simulink model "keyboardTask"  (R2012b)
settings: Solver=FixedStepDiscrete  StartTime=0.0  StopTime=10.0  FixedStep=0.001  RelTol=1e-3
undefined symbols (not defined in the file or in its folder): acquireMethods, autoplayMovementDuration, autoplayReactionTime, autoplayRotationDuration, autoplayRotationStart, centerOffset, clickPercentage, clickRefractoryPeriod, clickTargetColor, clickTargetHoverColor, cuedText, cuedTextLength, cumulativeDwell, cursorColorClick, cursorColorClosed, cursorColorOpen, cursorDiameter, cursorNeuralColor, cursorNonneuralColor, delayOrder, displayObject, displayShape, displayShape_1, displayShape_10, displayShape_11, displayShape_12, displayShape_13, displayShape_14, displayShape_15, displayShape_16, displayShape_17, displayShape_18, displayShape_19, displayShape_2, displayShape_3, displayShape_4, displayShape_5, displayShape_6, displayShape_7, displayShape_8, displayShape_9, dwellRefractoryPeriod, errorAssistAxis, errorAssistR, errorAssistTheta, expRandBinSize, expRandMax, expRandMin, expRandMu, failOnLiftoff, failurePenalty, falseClickFails, fingerPositionTolerance, fixedSeqMode, gain, gloveBias, gloveLPDenominator, gloveLPNumerator, gloveNonlinearCorrection, gloveXCorrection ... (+327)
(part 1 of 2)
settings Model: Creator=gilja  LastModifiedBy=NPTL
settings SolverCC: EnableConcurrentExecution=on  ConcurrentTasks=on
settings DataIOCC: SaveOutput=off  SignalLogging=off  SaveTime=off
settings OptimizationCC: InlineParams=on  InlineInvariantSignals=on  EnhancedBackFolding=on  EfficientFloat2IntCast=on  SimCompilerOptimization=On
settings DebuggingCC: UnderspecifiedInitializationDetection=Simplified
settings HardwareCC: ProdIntDivRoundTo=Zero  ProdEndianess=LittleEndian  ProdHWDeviceType=Generic->32-bit x86 compatible
settings RTWCC: SystemTargetFile=xpctarget.tlc  TemplateMakefile=xpc_default_tmf  Description=xPC Target  ProcessScript=xpctarget_make_rtw_hook  RTWCompilerOptimization=On
settings CodeAppCC: MaxIdLength=62
settings xpcTargetCC: TargetFcnLib=ansi_tfl_table_tmw.mat  CodeReplacementLibrary=XPC_BLAS  ParMdlRefBuildCompliant=on  ConcurrentExecutionCompliant=on  CombineSignalStateStructs=off  GRTInterface=on  xPCTaskExecutionProfile=on  xPCRL32EventNumber=5000  xPCisDownloadable=off  xPCLoadParamSetFile=off  xPCConcurrentTasks=off  xPCEnableSFAnimation=off

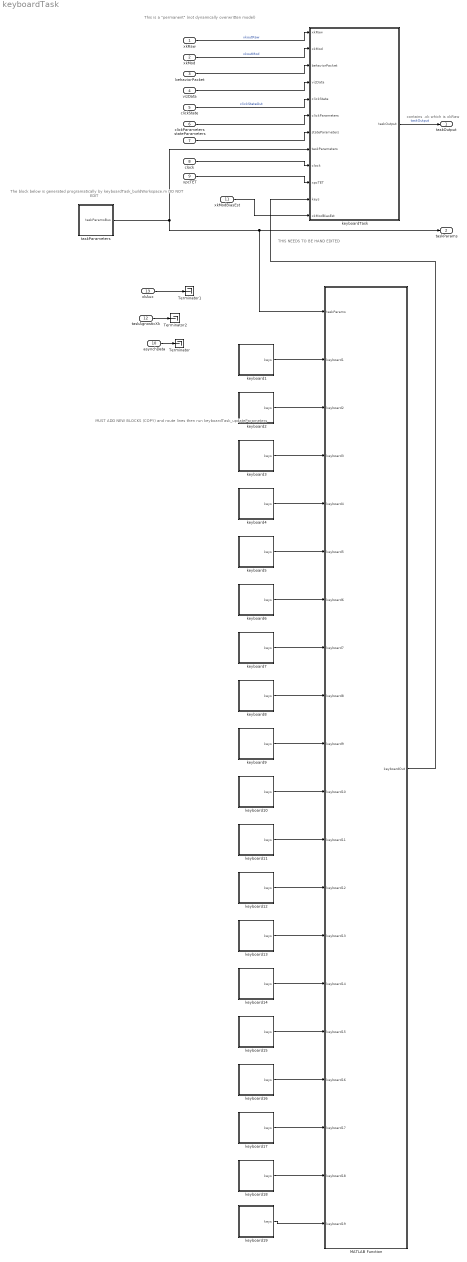
== system keyboardTask ==
  note: MUST ADD NEW BLOCKS (COPY)
      | and route lines
      | then run keyboardTask_updateParameters
  note: THIS NEEDS TO BE HAND EDITED
  note: contains .xk which is xkRaw
  note: The block below is generated programatically
      | by keyboardTask_buildWorkspace.m
      | DO NOT EDIT
  note: This is a "permanent" (not dynamically overwritten model)
  xkRaw : Inport  OutDataTypeStr=double  PortDimensions=[double(xkConstants.NUM_STATE_DIMENSIONS),1]  SampleTime=[0.001,0]
  xkMod : Inport  Port=2  OutDataTypeStr=double  PortDimensions=[double(xkConstants.NUM_STATE_DIMENSIONS),1]  SampleTime=[0.001,0]
  behaviorPacket : Inport  Port=3  OutDataTypeStr=Bus: behaviorPacketBus  SampleTime=[0.001,0]
  vizData : Inport  Port=4  OutDataTypeStr=Bus: peripheralData  SampleTime=[0.001,0]
  clickState : Inport  Port=5  OutDataTypeStr=uint16  PortDimensions=1  SampleTime=[0.001,0]
  clickParameters : Inport  Port=6  OutDataTypeStr=Bus: clickParametersBus  SampleTime=[0.001,0]
  stateParameters : Inport  Port=7  OutDataTypeStr=Bus: stateParams  SampleTime=[0.001,0]
  clock : Inport  Port=8  OutDataTypeStr=uint32  PortDimensions=1  SampleTime=[0.001,0]
  xpcTET : Inport  Port=9  OutDataTypeStr=double  PortDimensions=1  SampleTime=[0.001,0]
  asynchData : Inport  Port=10  OutDataTypeStr=Bus: peripheralData  SampleTime=[0.001,0]
  xkModBiasEst : Inport  Port=11  OutDataTypeStr=double  PortDimensions=[double(xkConstants.NUM_STATE_DIMENSIONS),1]  SampleTime=[0.001,0]
  taskAgnosticXk : Inport  Port=12  OutDataTypeStr=double  PortDimensions=[double(xkConstants.NUM_STATE_DIMENSIONS),1]  SampleTime=[0.001,0]
  xkAux : Inport  Port=13  OutDataTypeStr=double  PortDimensions=[double(xkConstants.NUM_STATE_DIMENSIONS),1]  SampleTime=[0.001,0]
  MATLAB Function : MATLAB Function  TreatAsAtomicUnit=on
  Terminator : Terminator
  Terminator1 : Terminator
  Terminator2 : Terminator
  keyboard1 : Subsystem
  keyboard10 : Subsystem
  keyboard11 : Subsystem
  keyboard12 : Subsystem
  keyboard13 : Subsystem
  keyboard14 : Subsystem
  keyboard15 : Subsystem
  keyboard16 : Subsystem
  keyboard17 : Subsystem
  keyboard18 : Subsystem
  keyboard19 : Subsystem
  keyboard2 : Subsystem
  keyboard3 : Subsystem
  keyboard4 : Subsystem
  keyboard5 : Subsystem
  keyboard6 : Subsystem
  keyboard7 : Subsystem
  keyboard8 : Subsystem
  keyboard9 : Subsystem
  keyboardTask : MATLAB Function  TreatAsAtomicUnit=on
  taskParameters : Subsystem
  taskOutput : Outport  OutDataTypeStr=Bus: taskOutput  PortDimensions=1  SampleTime=[0.001,0]  BusOutputAsStruct=on
  taskParams : Outport  Port=2  OutDataTypeStr=Bus: taskParamsBus  SampleTime=[0.001,0]
  wires:
  behaviorPacket/1 -> keyboardTask/3(behaviorPacket)
  vizData/1 -> keyboardTask/4(vizData)
  clickState/1 -> keyboardTask/5(clickState)  "clickStateOut"
  clickParameters/1 -> keyboardTask/6(clickParameters)
  clock/1 -> keyboardTask/9(clock)
  xpcTET/1 -> keyboardTask/10(xpcTET)
  keyboardTask/1(taskOutput) -> taskOutput/1  "taskOutput"
  stateParameters/1 -> keyboardTask/7(stateParameters)
  taskParameters/1(taskParamsBus) -> MATLAB Function/1(taskParams), taskParams/1, keyboardTask/8(taskParameters)
  MATLAB Function/1(keyboardOut) -> keyboardTask/11(keys)
  asynchData/1 -> Terminator/1
  xkRaw/1 -> keyboardTask/1(xkRaw)  "xkoutRaw"
  xkMod/1 -> keyboardTask/2(xkMod)  "xkoutMod"
  keyboard4/1(keys) -> MATLAB Function/5(keyboard4)
  keyboard3/1(keys) -> MATLAB Function/4(keyboard3)
  keyboard5/1(keys) -> MATLAB Function/6(keyboard5)
  keyboard2/1(keys) -> MATLAB Function/3(keyboard2)
  keyboard6/1(keys) -> MATLAB Function/7(keyboard6)
  keyboard7/1(keys) -> MATLAB Function/8(keyboard7)
  keyboard1/1(keys) -> MATLAB Function/2(keyboard1)
  keyboard8/1(keys) -> MATLAB Function/9(keyboard8)
  keyboard9/1(keys) -> MATLAB Function/10(keyboard9)
  keyboard10/1(keys) -> MATLAB Function/11(keyboard10)
  keyboard11/1(keys) -> MATLAB Function/12(keyboard11)
  keyboard12/1(keys) -> MATLAB Function/13(keyboard12)
  keyboard13/1(keys) -> MATLAB Function/14(keyboard13)
  keyboard14/1(keys) -> MATLAB Function/15(keyboard14)
  keyboard15/1(keys) -> MATLAB Function/16(keyboard15)
  keyboard16/1(keys) -> MATLAB Function/17(keyboard16)
  keyboard17/1(keys) -> MATLAB Function/18(keyboard17)
  keyboard18/1(keys) -> MATLAB Function/19(keyboard18)
  keyboard19/1(keys) -> MATLAB Function/20(keyboard19)
  xkAux/1 -> Terminator1/1
  taskAgnosticXk/1 -> Terminator2/1
  xkModBiasEst/1 -> keyboardTask/12(xkModBiasEst)

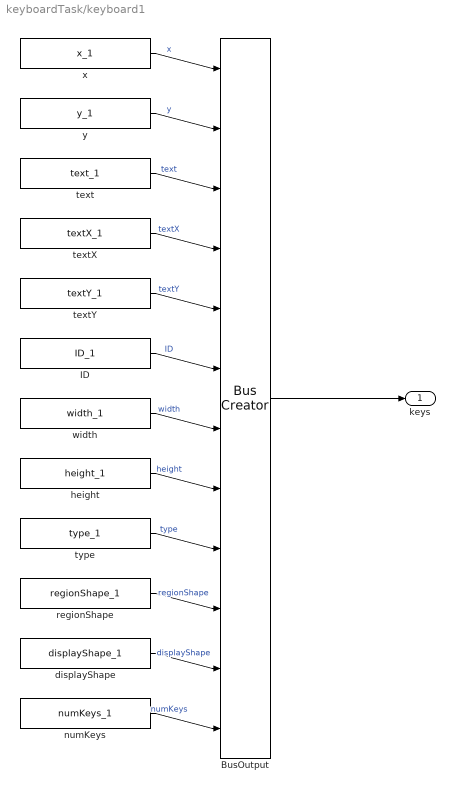
== system keyboardTask/keyboard1 ==
  BusOutput : BusCreator  Inputs=x,y,text,textX,textY,ID,width,height,type,regionShape,displayShape,numKeys  OutDataTypeStr=Bus: keysParamsBus
  ID : Constant  Value=ID_1
  displayShape : Constant  Value=displayShape_1
  height : Constant  Value=height_1
  numKeys : Constant  Value=numKeys_1
  regionShape : Constant  Value=regionShape_1
  text : Constant  Value=text_1
  textX : Constant  Value=textX_1
  textY : Constant  Value=textY_1
  type : Constant  Value=type_1
  width : Constant  Value=width_1
  x : Constant  Value=x_1
  y : Constant  Value=y_1
  keys : Outport
  wires:
  x/1 -> BusOutput/1  "x"
  y/1 -> BusOutput/2  "y"
  text/1 -> BusOutput/3  "text"
  textX/1 -> BusOutput/4  "textX"
  textY/1 -> BusOutput/5  "textY"
  ID/1 -> BusOutput/6  "ID"
  width/1 -> BusOutput/7  "width"
  height/1 -> BusOutput/8  "height"
  type/1 -> BusOutput/9  "type"
  regionShape/1 -> BusOutput/10  "regionShape"
  displayShape/1 -> BusOutput/11  "displayShape"
  numKeys/1 -> BusOutput/12  "numKeys"
  BusOutput/1 -> keys/1

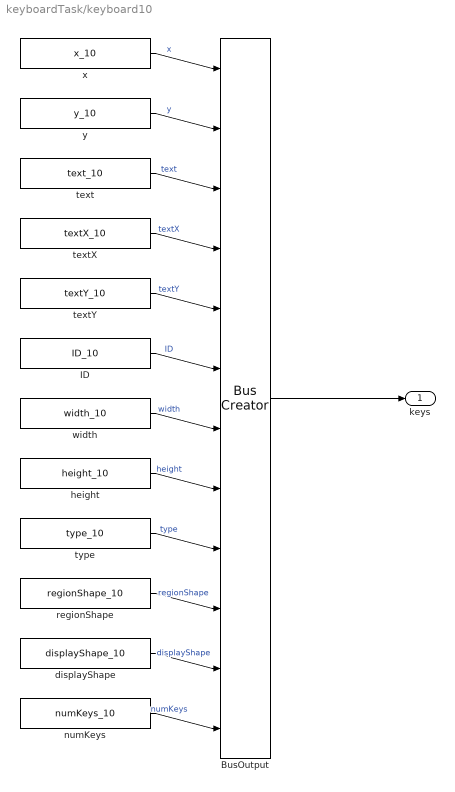
== system keyboardTask/keyboard10 ==
  BusOutput : BusCreator  Inputs=x,y,text,textX,textY,ID,width,height,type,regionShape,displayShape,numKeys  OutDataTypeStr=Bus: keysParamsBus
  ID : Constant  Value=ID_10
  displayShape : Constant  Value=displayShape_10
  height : Constant  Value=height_10
  numKeys : Constant  Value=numKeys_10
  regionShape : Constant  Value=regionShape_10
  text : Constant  Value=text_10
  textX : Constant  Value=textX_10
  textY : Constant  Value=textY_10
  type : Constant  Value=type_10
  width : Constant  Value=width_10
  x : Constant  Value=x_10
  y : Constant  Value=y_10
  keys : Outport  OutDataTypeStr=Bus: keysParamsBus
  wires:
  x/1 -> BusOutput/1  "x"
  y/1 -> BusOutput/2  "y"
  text/1 -> BusOutput/3  "text"
  textX/1 -> BusOutput/4  "textX"
  textY/1 -> BusOutput/5  "textY"
  ID/1 -> BusOutput/6  "ID"
  width/1 -> BusOutput/7  "width"
  height/1 -> BusOutput/8  "height"
  type/1 -> BusOutput/9  "type"
  regionShape/1 -> BusOutput/10  "regionShape"
  displayShape/1 -> BusOutput/11  "displayShape"
  numKeys/1 -> BusOutput/12  "numKeys"
  BusOutput/1 -> keys/1

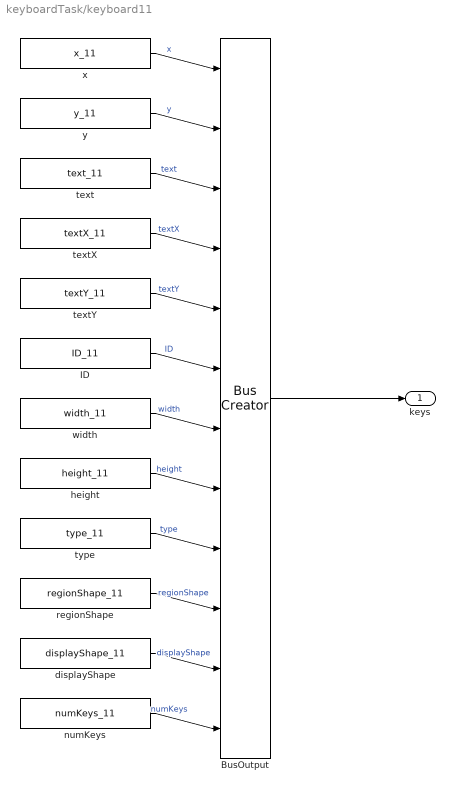
== system keyboardTask/keyboard11 ==
  BusOutput : BusCreator  Inputs=x,y,text,textX,textY,ID,width,height,type,regionShape,displayShape,numKeys  OutDataTypeStr=Bus: keysParamsBus
  ID : Constant  Value=ID_11
  displayShape : Constant  Value=displayShape_11
  height : Constant  Value=height_11
  numKeys : Constant  Value=numKeys_11
  regionShape : Constant  Value=regionShape_11
  text : Constant  Value=text_11
  textX : Constant  Value=textX_11
  textY : Constant  Value=textY_11
  type : Constant  Value=type_11
  width : Constant  Value=width_11
  x : Constant  Value=x_11
  y : Constant  Value=y_11
  keys : Outport  OutDataTypeStr=Bus: keysParamsBus
  wires:
  x/1 -> BusOutput/1  "x"
  y/1 -> BusOutput/2  "y"
  text/1 -> BusOutput/3  "text"
  textX/1 -> BusOutput/4  "textX"
  textY/1 -> BusOutput/5  "textY"
  ID/1 -> BusOutput/6  "ID"
  width/1 -> BusOutput/7  "width"
  height/1 -> BusOutput/8  "height"
  type/1 -> BusOutput/9  "type"
  regionShape/1 -> BusOutput/10  "regionShape"
  displayShape/1 -> BusOutput/11  "displayShape"
  numKeys/1 -> BusOutput/12  "numKeys"
  BusOutput/1 -> keys/1

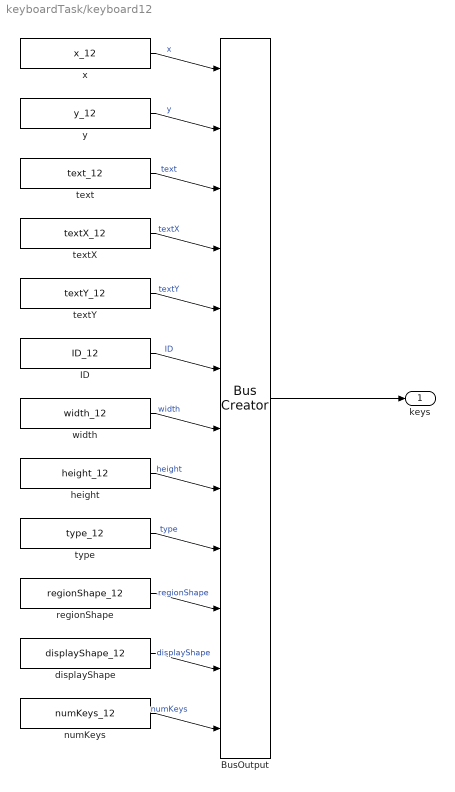
== system keyboardTask/keyboard12 ==
  BusOutput : BusCreator  Inputs=x,y,text,textX,textY,ID,width,height,type,regionShape,displayShape,numKeys  OutDataTypeStr=Bus: keysParamsBus
  ID : Constant  Value=ID_12
  displayShape : Constant  Value=displayShape_12
  height : Constant  Value=height_12
  numKeys : Constant  Value=numKeys_12
  regionShape : Constant  Value=regionShape_12
  text : Constant  Value=text_12
  textX : Constant  Value=textX_12
  textY : Constant  Value=textY_12
  type : Constant  Value=type_12
  width : Constant  Value=width_12
  x : Constant  Value=x_12
  y : Constant  Value=y_12
  keys : Outport  OutDataTypeStr=Bus: keysParamsBus
  wires:
  x/1 -> BusOutput/1  "x"
  y/1 -> BusOutput/2  "y"
  text/1 -> BusOutput/3  "text"
  textX/1 -> BusOutput/4  "textX"
  textY/1 -> BusOutput/5  "textY"
  ID/1 -> BusOutput/6  "ID"
  width/1 -> BusOutput/7  "width"
  height/1 -> BusOutput/8  "height"
  type/1 -> BusOutput/9  "type"
  regionShape/1 -> BusOutput/10  "regionShape"
  displayShape/1 -> BusOutput/11  "displayShape"
  numKeys/1 -> BusOutput/12  "numKeys"
  BusOutput/1 -> keys/1

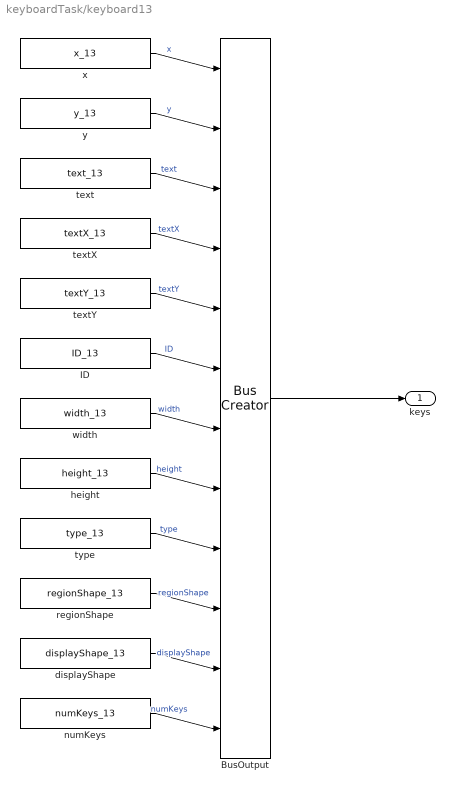
== system keyboardTask/keyboard13 ==
  BusOutput : BusCreator  Inputs=x,y,text,textX,textY,ID,width,height,type,regionShape,displayShape,numKeys  OutDataTypeStr=Bus: keysParamsBus
  ID : Constant  Value=ID_13
  displayShape : Constant  Value=displayShape_13
  height : Constant  Value=height_13
  numKeys : Constant  Value=numKeys_13
  regionShape : Constant  Value=regionShape_13
  text : Constant  Value=text_13
  textX : Constant  Value=textX_13
  textY : Constant  Value=textY_13
  type : Constant  Value=type_13
  width : Constant  Value=width_13
  x : Constant  Value=x_13
  y : Constant  Value=y_13
  keys : Outport  OutDataTypeStr=Bus: keysParamsBus
  wires:
  x/1 -> BusOutput/1  "x"
  y/1 -> BusOutput/2  "y"
  text/1 -> BusOutput/3  "text"
  textX/1 -> BusOutput/4  "textX"
  textY/1 -> BusOutput/5  "textY"
  ID/1 -> BusOutput/6  "ID"
  width/1 -> BusOutput/7  "width"
  height/1 -> BusOutput/8  "height"
  type/1 -> BusOutput/9  "type"
  regionShape/1 -> BusOutput/10  "regionShape"
  displayShape/1 -> BusOutput/11  "displayShape"
  numKeys/1 -> BusOutput/12  "numKeys"
  BusOutput/1 -> keys/1

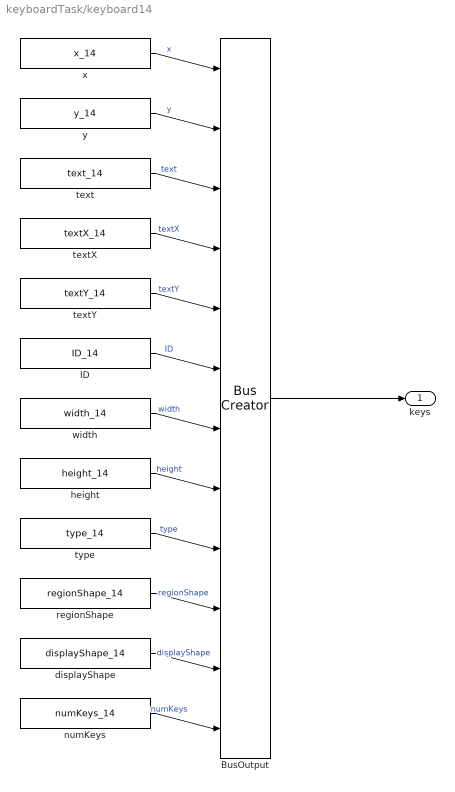
== system keyboardTask/keyboard14 ==
  BusOutput : BusCreator  Inputs=x,y,text,textX,textY,ID,width,height,type,regionShape,displayShape,numKeys  OutDataTypeStr=Bus: keysParamsBus
  ID : Constant  Value=ID_14
  displayShape : Constant  Value=displayShape_14
  height : Constant  Value=height_14
  numKeys : Constant  Value=numKeys_14
  regionShape : Constant  Value=regionShape_14
  text : Constant  Value=text_14
  textX : Constant  Value=textX_14
  textY : Constant  Value=textY_14
  type : Constant  Value=type_14
  width : Constant  Value=width_14
  x : Constant  Value=x_14
  y : Constant  Value=y_14
  keys : Outport  OutDataTypeStr=Bus: keysParamsBus
  wires:
  x/1 -> BusOutput/1  "x"
  y/1 -> BusOutput/2  "y"
  text/1 -> BusOutput/3  "text"
  textX/1 -> BusOutput/4  "textX"
  textY/1 -> BusOutput/5  "textY"
  ID/1 -> BusOutput/6  "ID"
  width/1 -> BusOutput/7  "width"
  height/1 -> BusOutput/8  "height"
  type/1 -> BusOutput/9  "type"
  regionShape/1 -> BusOutput/10  "regionShape"
  displayShape/1 -> BusOutput/11  "displayShape"
  numKeys/1 -> BusOutput/12  "numKeys"
  BusOutput/1 -> keys/1

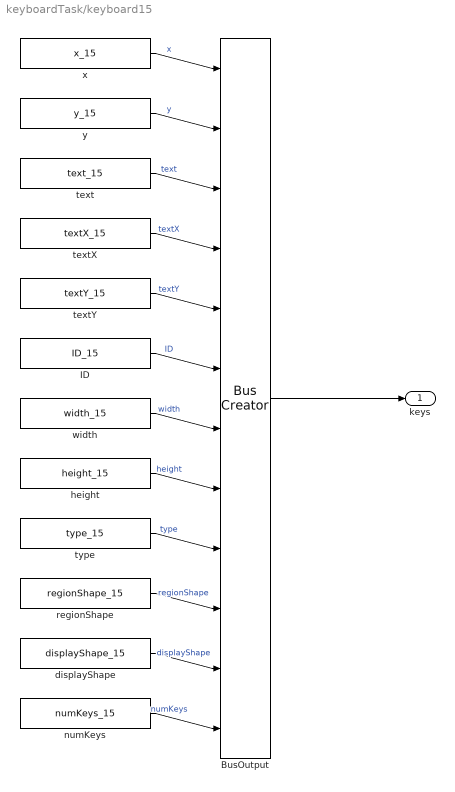
== system keyboardTask/keyboard15 ==
  BusOutput : BusCreator  Inputs=x,y,text,textX,textY,ID,width,height,type,regionShape,displayShape,numKeys  OutDataTypeStr=Bus: keysParamsBus
  ID : Constant  Value=ID_15
  displayShape : Constant  Value=displayShape_15
  height : Constant  Value=height_15
  numKeys : Constant  Value=numKeys_15
  regionShape : Constant  Value=regionShape_15
  text : Constant  Value=text_15
  textX : Constant  Value=textX_15
  textY : Constant  Value=textY_15
  type : Constant  Value=type_15
  width : Constant  Value=width_15
  x : Constant  Value=x_15
  y : Constant  Value=y_15
  keys : Outport  OutDataTypeStr=Bus: keysParamsBus
  wires:
  x/1 -> BusOutput/1  "x"
  y/1 -> BusOutput/2  "y"
  text/1 -> BusOutput/3  "text"
  textX/1 -> BusOutput/4  "textX"
  textY/1 -> BusOutput/5  "textY"
  ID/1 -> BusOutput/6  "ID"
  width/1 -> BusOutput/7  "width"
  height/1 -> BusOutput/8  "height"
  type/1 -> BusOutput/9  "type"
  regionShape/1 -> BusOutput/10  "regionShape"
  displayShape/1 -> BusOutput/11  "displayShape"
  numKeys/1 -> BusOutput/12  "numKeys"
  BusOutput/1 -> keys/1

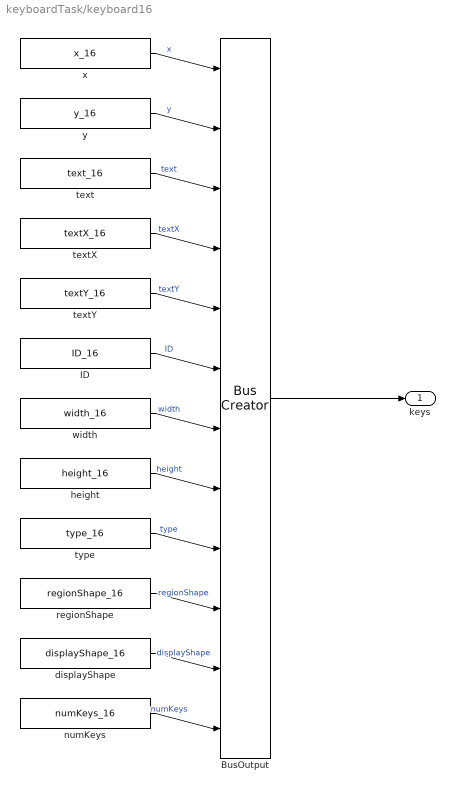
== system keyboardTask/keyboard16 ==
  BusOutput : BusCreator  Inputs=x,y,text,textX,textY,ID,width,height,type,regionShape,displayShape,numKeys  OutDataTypeStr=Bus: keysParamsBus
  ID : Constant  Value=ID_16
  displayShape : Constant  Value=displayShape_16
  height : Constant  Value=height_16
  numKeys : Constant  Value=numKeys_16
  regionShape : Constant  Value=regionShape_16
  text : Constant  Value=text_16
  textX : Constant  Value=textX_16
  textY : Constant  Value=textY_16
  type : Constant  Value=type_16
  width : Constant  Value=width_16
  x : Constant  Value=x_16
  y : Constant  Value=y_16
  keys : Outport  OutDataTypeStr=Bus: keysParamsBus
  wires:
  x/1 -> BusOutput/1  "x"
  y/1 -> BusOutput/2  "y"
  text/1 -> BusOutput/3  "text"
  textX/1 -> BusOutput/4  "textX"
  textY/1 -> BusOutput/5  "textY"
  ID/1 -> BusOutput/6  "ID"
  width/1 -> BusOutput/7  "width"
  height/1 -> BusOutput/8  "height"
  type/1 -> BusOutput/9  "type"
  regionShape/1 -> BusOutput/10  "regionShape"
  displayShape/1 -> BusOutput/11  "displayShape"
  numKeys/1 -> BusOutput/12  "numKeys"
  BusOutput/1 -> keys/1

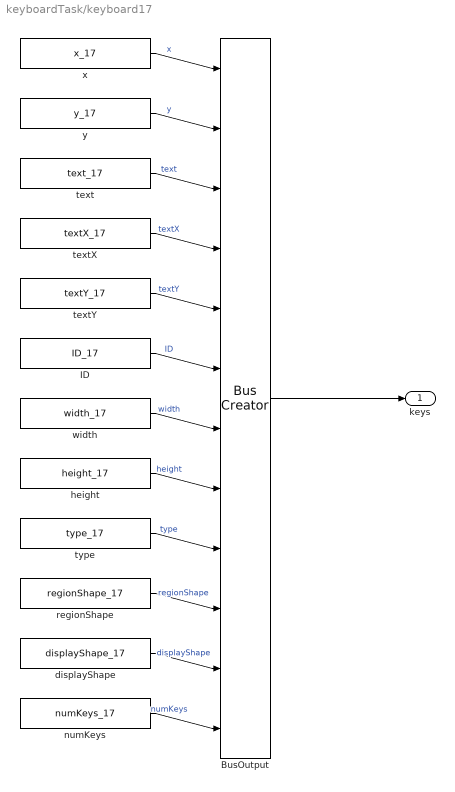
== system keyboardTask/keyboard17 ==
  BusOutput : BusCreator  Inputs=x,y,text,textX,textY,ID,width,height,type,regionShape,displayShape,numKeys  OutDataTypeStr=Bus: keysParamsBus
  ID : Constant  Value=ID_17
  displayShape : Constant  Value=displayShape_17
  height : Constant  Value=height_17
  numKeys : Constant  Value=numKeys_17
  regionShape : Constant  Value=regionShape_17
  text : Constant  Value=text_17
  textX : Constant  Value=textX_17
  textY : Constant  Value=textY_17
  type : Constant  Value=type_17
  width : Constant  Value=width_17
  x : Constant  Value=x_17
  y : Constant  Value=y_17
  keys : Outport  OutDataTypeStr=Bus: keysParamsBus
  wires:
  x/1 -> BusOutput/1  "x"
  y/1 -> BusOutput/2  "y"
  text/1 -> BusOutput/3  "text"
  textX/1 -> BusOutput/4  "textX"
  textY/1 -> BusOutput/5  "textY"
  ID/1 -> BusOutput/6  "ID"
  width/1 -> BusOutput/7  "width"
  height/1 -> BusOutput/8  "height"
  type/1 -> BusOutput/9  "type"
  regionShape/1 -> BusOutput/10  "regionShape"
  displayShape/1 -> BusOutput/11  "displayShape"
  numKeys/1 -> BusOutput/12  "numKeys"
  BusOutput/1 -> keys/1

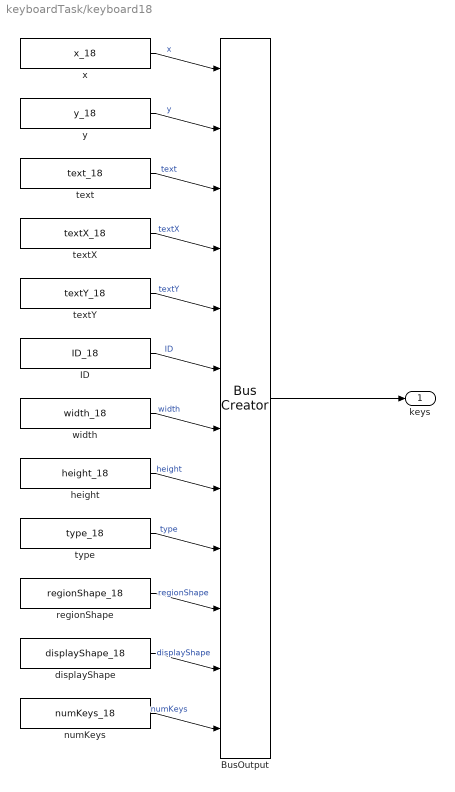
== system keyboardTask/keyboard18 ==
  BusOutput : BusCreator  Inputs=x,y,text,textX,textY,ID,width,height,type,regionShape,displayShape,numKeys  OutDataTypeStr=Bus: keysParamsBus
  ID : Constant  Value=ID_18
  displayShape : Constant  Value=displayShape_18
  height : Constant  Value=height_18
  numKeys : Constant  Value=numKeys_18
  regionShape : Constant  Value=regionShape_18
  text : Constant  Value=text_18
  textX : Constant  Value=textX_18
  textY : Constant  Value=textY_18
  type : Constant  Value=type_18
  width : Constant  Value=width_18
  x : Constant  Value=x_18
  y : Constant  Value=y_18
  keys : Outport  OutDataTypeStr=Bus: keysParamsBus
  wires:
  x/1 -> BusOutput/1  "x"
  y/1 -> BusOutput/2  "y"
  text/1 -> BusOutput/3  "text"
  textX/1 -> BusOutput/4  "textX"
  textY/1 -> BusOutput/5  "textY"
  ID/1 -> BusOutput/6  "ID"
  width/1 -> BusOutput/7  "width"
  height/1 -> BusOutput/8  "height"
  type/1 -> BusOutput/9  "type"
  regionShape/1 -> BusOutput/10  "regionShape"
  displayShape/1 -> BusOutput/11  "displayShape"
  numKeys/1 -> BusOutput/12  "numKeys"
  BusOutput/1 -> keys/1

== system keyboardTask/keyboard19 ==
  BusOutput : BusCreator  Inputs=x,y,text,textX,textY,ID,width,height,type,regionShape,displayShape,numKeys  OutDataTypeStr=Bus: keysParamsBus
  ID : Constant  Value=ID_19
  displayShape : Constant  Value=displayShape_19
  height : Constant  Value=height_19
  numKeys : Constant  Value=numKeys_19
  regionShape : Constant  Value=regionShape_19
  text : Constant  Value=text_19
  textX : Constant  Value=textX_19
  textY : Constant  Value=textY_19
  type : Constant  Value=type_19
  width : Constant  Value=width_19
  x : Constant  Value=x_19
  y : Constant  Value=y_19
  keys : Outport  OutDataTypeStr=Bus: keysParamsBus
  wires:
  x/1 -> BusOutput/1  "x"
  y/1 -> BusOutput/2  "y"
  text/1 -> BusOutput/3  "text"
  textX/1 -> BusOutput/4  "textX"
  textY/1 -> BusOutput/5  "textY"
  ID/1 -> BusOutput/6  "ID"
  width/1 -> BusOutput/7  "width"
  height/1 -> BusOutput/8  "height"
  type/1 -> BusOutput/9  "type"
  regionShape/1 -> BusOutput/10  "regionShape"
  displayShape/1 -> BusOutput/11  "displayShape"
  numKeys/1 -> BusOutput/12  "numKeys"
  BusOutput/1 -> keys/1

== system keyboardTask/keyboard2 ==
  BusOutput : BusCreator  Inputs=x,y,text,textX,textY,ID,width,height,type,regionShape,displayShape,numKeys  OutDataTypeStr=Bus: keysParamsBus
  ID : Constant  Value=ID_2
  displayShape : Constant  Value=displayShape_2
  height : Constant  Value=height_2
  numKeys : Constant  Value=numKeys_2
  regionShape : Constant  Value=regionShape_2
  text : Constant  Value=text_2
  textX : Constant  Value=textX_2
  textY : Constant  Value=textY_2
  type : Constant  Value=type_2
  width : Constant  Value=width_2
  x : Constant  Value=x_2
  y : Constant  Value=y_2
  keys : Outport  OutDataTypeStr=Bus: keysParamsBus
  wires:
  x/1 -> BusOutput/1  "x"
  y/1 -> BusOutput/2  "y"
  text/1 -> BusOutput/3  "text"
  textX/1 -> BusOutput/4  "textX"
  textY/1 -> BusOutput/5  "textY"
  ID/1 -> BusOutput/6  "ID"
  width/1 -> BusOutput/7  "width"
  height/1 -> BusOutput/8  "height"
  type/1 -> BusOutput/9  "type"
  regionShape/1 -> BusOutput/10  "regionShape"
  displayShape/1 -> BusOutput/11  "displayShape"
  numKeys/1 -> BusOutput/12  "numKeys"
  BusOutput/1 -> keys/1

== system keyboardTask/keyboard3 ==
  BusOutput : BusCreator  Inputs=x,y,text,textX,textY,ID,width,height,type,regionShape,displayShape,numKeys  OutDataTypeStr=Bus: keysParamsBus
  ID : Constant  Value=ID_3
  displayShape : Constant  Value=displayShape_3
  height : Constant  Value=height_3
  numKeys : Constant  Value=numKeys_3
  regionShape : Constant  Value=regionShape_3
  text : Constant  Value=text_3
  textX : Constant  Value=textX_3
  textY : Constant  Value=textY_3
  type : Constant  Value=type_3
  width : Constant  Value=width_3
  x : Constant  Value=x_3
  y : Constant  Value=y_3
  keys : Outport  OutDataTypeStr=Bus: keysParamsBus
  wires:
  x/1 -> BusOutput/1  "x"
  y/1 -> BusOutput/2  "y"
  text/1 -> BusOutput/3  "text"
  textX/1 -> BusOutput/4  "textX"
  textY/1 -> BusOutput/5  "textY"
  ID/1 -> BusOutput/6  "ID"
  width/1 -> BusOutput/7  "width"
  height/1 -> BusOutput/8  "height"
  type/1 -> BusOutput/9  "type"
  regionShape/1 -> BusOutput/10  "regionShape"
  displayShape/1 -> BusOutput/11  "displayShape"
  numKeys/1 -> BusOutput/12  "numKeys"
  BusOutput/1 -> keys/1

== system keyboardTask/keyboard4 ==
  BusOutput : BusCreator  Inputs=x,y,text,textX,textY,ID,width,height,type,regionShape,displayShape,numKeys  OutDataTypeStr=Bus: keysParamsBus
  ID : Constant  Value=ID_4
  displayShape : Constant  Value=displayShape_4
  height : Constant  Value=height_4
  numKeys : Constant  Value=numKeys_4
  regionShape : Constant  Value=regionShape_4
  text : Constant  Value=text_4
  textX : Constant  Value=textX_4
  textY : Constant  Value=textY_4
  type : Constant  Value=type_4
  width : Constant  Value=width_4
  x : Constant  Value=x_4
  y : Constant  Value=y_4
  keys : Outport  OutDataTypeStr=Bus: keysParamsBus
  wires:
  x/1 -> BusOutput/1  "x"
  y/1 -> BusOutput/2  "y"
  text/1 -> BusOutput/3  "text"
  textX/1 -> BusOutput/4  "textX"
  textY/1 -> BusOutput/5  "textY"
  ID/1 -> BusOutput/6  "ID"
  width/1 -> BusOutput/7  "width"
  height/1 -> BusOutput/8  "height"
  type/1 -> BusOutput/9  "type"
  regionShape/1 -> BusOutput/10  "regionShape"
  displayShape/1 -> BusOutput/11  "displayShape"
  numKeys/1 -> BusOutput/12  "numKeys"
  BusOutput/1 -> keys/1

== system keyboardTask/keyboard5 ==
  BusOutput : BusCreator  Inputs=x,y,text,textX,textY,ID,width,height,type,regionShape,displayShape,numKeys  OutDataTypeStr=Bus: keysParamsBus
  ID : Constant  Value=ID_5
  displayShape : Constant  Value=displayShape_5
  height : Constant  Value=height_5
  numKeys : Constant  Value=numKeys_5
  regionShape : Constant  Value=regionShape_5
  text : Constant  Value=text_5
  textX : Constant  Value=textX_5
  textY : Constant  Value=textY_5
  type : Constant  Value=type_5
  width : Constant  Value=width_5
  x : Constant  Value=x_5
  y : Constant  Value=y_5
  keys : Outport  OutDataTypeStr=Bus: keysParamsBus
  wires:
  x/1 -> BusOutput/1  "x"
  y/1 -> BusOutput/2  "y"
  text/1 -> BusOutput/3  "text"
  textX/1 -> BusOutput/4  "textX"
  textY/1 -> BusOutput/5  "textY"
  ID/1 -> BusOutput/6  "ID"
  width/1 -> BusOutput/7  "width"
  height/1 -> BusOutput/8  "height"
  type/1 -> BusOutput/9  "type"
  regionShape/1 -> BusOutput/10  "regionShape"
  displayShape/1 -> BusOutput/11  "displayShape"
  numKeys/1 -> BusOutput/12  "numKeys"
  BusOutput/1 -> keys/1

== system keyboardTask/keyboard6 ==
  BusOutput : BusCreator  Inputs=x,y,text,textX,textY,ID,width,height,type,regionShape,displayShape,numKeys  OutDataTypeStr=Bus: keysParamsBus
  ID : Constant  Value=ID_6
  displayShape : Constant  Value=displayShape_6
  height : Constant  Value=height_6
  numKeys : Constant  Value=numKeys_6
  regionShape : Constant  Value=regionShape_6
  text : Constant  Value=text_6
  textX : Constant  Value=textX_6
  textY : Constant  Value=textY_6
  type : Constant  Value=type_6
  width : Constant  Value=width_6
  x : Constant  Value=x_6
  y : Constant  Value=y_6
  keys : Outport  OutDataTypeStr=Bus: keysParamsBus
  wires:
  x/1 -> BusOutput/1  "x"
  y/1 -> BusOutput/2  "y"
  text/1 -> BusOutput/3  "text"
  textX/1 -> BusOutput/4  "textX"
  textY/1 -> BusOutput/5  "textY"
  ID/1 -> BusOutput/6  "ID"
  width/1 -> BusOutput/7  "width"
  height/1 -> BusOutput/8  "height"
  type/1 -> BusOutput/9  "type"
  regionShape/1 -> BusOutput/10  "regionShape"
  displayShape/1 -> BusOutput/11  "displayShape"
  numKeys/1 -> BusOutput/12  "numKeys"
  BusOutput/1 -> keys/1

== system keyboardTask/keyboard7 ==
  BusOutput : BusCreator  Inputs=x,y,text,textX,textY,ID,width,height,type,regionShape,displayShape,numKeys  OutDataTypeStr=Bus: keysParamsBus
  ID : Constant  Value=ID_7
  displayShape : Constant  Value=displayShape_7
  height : Constant  Value=height_7
  numKeys : Constant  Value=numKeys_7
  regionShape : Constant  Value=regionShape_7
  text : Constant  Value=text_7
  textX : Constant  Value=textX_7
  textY : Constant  Value=textY_7
  type : Constant  Value=type_7
  width : Constant  Value=width_7
  x : Constant  Value=x_7
  y : Constant  Value=y_7
  keys : Outport  OutDataTypeStr=Bus: keysParamsBus
  wires:
  x/1 -> BusOutput/1  "x"
  y/1 -> BusOutput/2  "y"
  text/1 -> BusOutput/3  "text"
  textX/1 -> BusOutput/4  "textX"
  textY/1 -> BusOutput/5  "textY"
  ID/1 -> BusOutput/6  "ID"
  width/1 -> BusOutput/7  "width"
  height/1 -> BusOutput/8  "height"
  type/1 -> BusOutput/9  "type"
  regionShape/1 -> BusOutput/10  "regionShape"
  displayShape/1 -> BusOutput/11  "displayShape"
  numKeys/1 -> BusOutput/12  "numKeys"
  BusOutput/1 -> keys/1

== system keyboardTask/keyboard8 ==
  BusOutput : BusCreator  Inputs=x,y,text,textX,textY,ID,width,height,type,regionShape,displayShape,numKeys  OutDataTypeStr=Bus: keysParamsBus
  ID : Constant  Value=ID_8
  displayShape : Constant  Value=displayShape_8
  height : Constant  Value=height_8
  numKeys : Constant  Value=numKeys_8
  regionShape : Constant  Value=regionShape_8
  text : Constant  Value=text_8
  textX : Constant  Value=textX_8
  textY : Constant  Value=textY_8
  type : Constant  Value=type_8
  width : Constant  Value=width_8
  x : Constant  Value=x_8
  y : Constant  Value=y_8
  keys : Outport  OutDataTypeStr=Bus: keysParamsBus
  wires:
  x/1 -> BusOutput/1  "x"
  y/1 -> BusOutput/2  "y"
  text/1 -> BusOutput/3  "text"
  textX/1 -> BusOutput/4  "textX"
  textY/1 -> BusOutput/5  "textY"
  ID/1 -> BusOutput/6  "ID"
  width/1 -> BusOutput/7  "width"
  height/1 -> BusOutput/8  "height"
  type/1 -> BusOutput/9  "type"
  regionShape/1 -> BusOutput/10  "regionShape"
  displayShape/1 -> BusOutput/11  "displayShape"
  numKeys/1 -> BusOutput/12  "numKeys"
  BusOutput/1 -> keys/1

== system keyboardTask/keyboard9 ==
  BusOutput : BusCreator  Inputs=x,y,text,textX,textY,ID,width,height,type,regionShape,displayShape,numKeys  OutDataTypeStr=Bus: keysParamsBus
  ID : Constant  Value=ID_9
  displayShape : Constant  Value=displayShape_9
  height : Constant  Value=height_9
  numKeys : Constant  Value=numKeys_9
  regionShape : Constant  Value=regionShape_9
  text : Constant  Value=text_9
  textX : Constant  Value=textX_9
  textY : Constant  Value=textY_9
  type : Constant  Value=type_9
  width : Constant  Value=width_9
  x : Constant  Value=x_9
  y : Constant  Value=y_9
  keys : Outport  OutDataTypeStr=Bus: keysParamsBus
  wires:
  x/1 -> BusOutput/1  "x"
  y/1 -> BusOutput/2  "y"
  text/1 -> BusOutput/3  "text"
  textX/1 -> BusOutput/4  "textX"
  textY/1 -> BusOutput/5  "textY"
  ID/1 -> BusOutput/6  "ID"
  width/1 -> BusOutput/7  "width"
  height/1 -> BusOutput/8  "height"
  type/1 -> BusOutput/9  "type"
  regionShape/1 -> BusOutput/10  "regionShape"
  displayShape/1 -> BusOutput/11  "displayShape"
  numKeys/1 -> BusOutput/12  "numKeys"
  BusOutput/1 -> keys/1

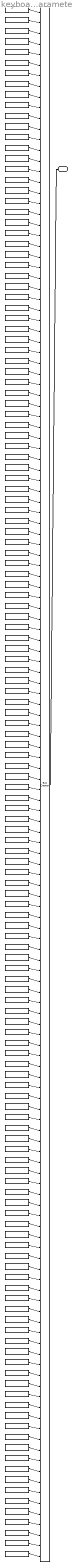
== system keyboardTask/taskParameters ==
  BusOutput : BusCreator  Inputs=targetDiameter,maxTaskTime,holdTime,trialTimeout,numTrials,randomSeed,expRandMu,expRandMin,expRandMax,expRandBinSize,taskType,targetInds,numTargets,gain,failurePenalty,cursorDiameter,inputType,gloveBias,useRandomDelay,mouseOffset,workspaceX,workspaceY,workspaceZ,workspaceR,workspaceR2,showScores,trialsPerScore,cursorColorClick,recenterOnFail,recenterOnSuccess,recenterDelay,initialInput,clickPercentage,lockFingerPosition,fingerPositionTolerance,failOnLiftoff,errorAssistR,errorAssistTheta,errorAssistAxis,useGloveLPF,gloveLPNumerator,gloveLPDenominator,gloveNonlinearCorrection,gloveYCorrection,gloveXCorrection,useMouseLPF,soundOnFail,soundOnGo,soundOnSuccess,soundOnOverTarget,mouseLPNumerator,mouseLPDenominator,stopOffTarget,stopOnClick,outputType,xk2HorizontalPos,xk2HorizontalVel,xk2VerticalPos,xk2VerticalVel,xk2DepthPos,xk2DepthVel,xk2RotatePos,xk2RotateVel,xk2Rotate2Pos,xk2Rotate2Vel,gridEdges,gridTilesEachDim,selectionRefractoryMS,autoplayReactionTime,autoplayMovementDuration,powerGain,powerGainUnityCrossing,targetRotDiameter,autoplayRotationStart,autoplayRotationDuration,randomTaskTargetDiameters,randomTaskTargetRotDiameters,randomTaskBoundaries,numDisplayDims,cursorColorOpen,cursorColorClosed,showXYZaura,displayObject,preTrialLength,targetDiameters,numTargetDiameters,minTargetDistance,targetDelay,targetSpaceX,targetSpaceY,clickTargetColor,clickTargetHoverColor,falseClickFails,splitDimensions,vmrTheta,xkRawSpeedCap,movementDuration,holdDuration,restDuration,returnDuration,repsPerBlock,whichMovements,movementOrder,delayOrder,clickRefractoryPeriod,xpcVelocityOutputPeriodMS,outputVelocityScaling,screenUpdateRate,targetDevice,playSpokenCues,numTargetsInSeq,targetSeq,seqReadyTime,seqRehearseTime,rotateSeqCues,numRepsPerSeq,rehearsalOrder,rehearsalTimes,pathMode,memorizeMode,fixedSeqMode,sequenceMatrix,keyboard,resetDisplay,cursorNeuralColor,cursorNonneuralColor,centerOffset,scoreTime,cuedTextLength,cuedText,keyboardDims,recenterFullscreen,soundOnError,acquireMethods,cumulativeDwell,showBackspace,showStartStop,showTargetText,showTypedText,showCueOnTarget,showCueOffTarget,recenterOffset,dwellRefractoryPeriod,keyPressedTime,initialLockout,initialState  OutDataTypeStr=Bus: taskParamsBus
  acquireMethods : Constant  Value=acquireMethods
  autoplayMovementDuration : Constant  Value=autoplayMovementDuration
  autoplayReactionTime : Constant  Value=autoplayReactionTime
  autoplayRotationDuration : Constant  Value=autoplayRotationDuration
  autoplayRotationStart : Constant  Value=autoplayRotationStart
  centerOffset : Constant  Value=centerOffset
  clickPercentage : Constant  Value=clickPercentage
  clickRefractoryPeriod : Constant  Value=clickRefractoryPeriod
  clickTargetColor : Constant  Value=clickTargetColor
  clickTargetHoverColor : Constant  Value=clickTargetHoverColor
  cuedText : Constant  Value=cuedText
  cuedTextLength : Constant  Value=cuedTextLength
  cumulativeDwell : Constant  Value=cumulativeDwell
  cursorColorClick : Constant  Value=cursorColorClick
  cursorColorClosed : Constant  Value=cursorColorClosed
  cursorColorOpen : Constant  Value=cursorColorOpen
  cursorDiameter : Constant  Value=cursorDiameter
  cursorNeuralColor : Constant  Value=cursorNeuralColor
  cursorNonneuralColor : Constant  Value=cursorNonneuralColor
  delayOrder : Constant  Value=delayOrder
  displayObject : Constant  Value=displayObject
  dwellRefractoryPeriod : Constant  Value=dwellRefractoryPeriod
  errorAssistAxis : Constant  Value=errorAssistAxis
  errorAssistR : Constant  Value=errorAssistR
  errorAssistTheta : Constant  Value=errorAssistTheta
  expRandBinSize : Constant  Value=expRandBinSize
  expRandMax : Constant  Value=expRandMax
  expRandMin : Constant  Value=expRandMin
  expRandMu : Constant  Value=expRandMu
  failOnLiftoff : Constant  Value=failOnLiftoff
  failurePenalty : Constant  Value=failurePenalty
  falseClickFails : Constant  Value=falseClickFails
  fingerPositionTolerance : Constant  Value=fingerPositionTolerance
  fixedSeqMode : Constant  Value=fixedSeqMode
  gain : Constant  Value=gain
  gloveBias : Constant  Value=gloveBias
  gloveLPDenominator : Constant  Value=gloveLPDenominator
  gloveLPNumerator : Constant  Value=gloveLPNumerator
  gloveNonlinearCorrection : Constant  Value=gloveNonlinearCorrection
  gloveXCorrection : Constant  Value=gloveXCorrection
  gloveYCorrection : Constant  Value=gloveYCorrection
  gridEdges : Constant  Value=gridEdges
  gridTilesEachDim : Constant  Value=gridTilesEachDim
  holdDuration : Constant  Value=holdDuration
  holdTime : Constant  Value=holdTime
  initialInput : Constant  Value=initialInput
  initialLockout : Constant  Value=initialLockout
  initialState : Constant  Value=initialState
  inputType : Constant  Value=inputType
  keyPressedTime : Constant  Value=keyPressedTime
  keyboard : Constant  Value=keyboard
  keyboardDims : Constant  Value=keyboardDims
  lockFingerPosition : Constant  Value=lockFingerPosition
  maxTaskTime : Constant  Value=maxTaskTime
  memorizeMode : Constant  Value=memorizeMode
  minTargetDistance : Constant  Value=minTargetDistance
  mouseLPDenominator : Constant  Value=mouseLPDenominator
  mouseLPNumerator : Constant  Value=mouseLPNumerator
  mouseOffset : Constant  Value=mouseOffset
  movementDuration : Constant  Value=movementDuration
  movementOrder : Constant  Value=movementOrder
  numDisplayDims : Constant  Value=numDisplayDims
  numRepsPerSeq : Constant  Value=numRepsPerSeq
  numTargetDiameters : Constant  Value=numTargetDiameters
  numTargets : Constant  Value=numTargets
  numTargetsInSeq : Constant  Value=numTargetsInSeq
  numTrials : Constant  Value=numTrials
  outputType : Constant  Value=outputType
  outputVelocityScaling : Constant  Value=outputVelocityScaling
  pathMode : Constant  Value=pathMode
  playSpokenCues : Constant  Value=playSpokenCues
  powerGain : Constant  Value=powerGain
  powerGainUnityCrossing : Constant  Value=powerGainUnityCrossing
  preTrialLength : Constant  Value=preTrialLength
  randomSeed : Constant  Value=randomSeed
  randomTaskBoundaries : Constant  Value=randomTaskBoundaries
  randomTaskTargetDiameters : Constant  Value=randomTaskTargetDiameters
  randomTaskTargetRotDiameters : Constant  Value=randomTaskTargetRotDiameters
  recenterDelay : Constant  Value=recenterDelay
  recenterFullscreen : Constant  Value=recenterFullscreen
  recenterOffset : Constant  Value=recenterOffset
  recenterOnFail : Constant  Value=recenterOnFail
  recenterOnSuccess : Constant  Value=recenterOnSuccess
  rehearsalOrder : Constant  Value=rehearsalOrder
  rehearsalTimes : Constant  Value=rehearsalTimes
  repsPerBlock : Constant  Value=repsPerBlock
  resetDisplay : Constant  Value=resetDisplay
  restDuration : Constant  Value=restDuration
  returnDuration : Constant  Value=returnDuration
  rotateSeqCues : Constant  Value=rotateSeqCues
  scoreTime : Constant  Value=scoreTime
  screenUpdateRate : Constant  Value=screenUpdateRate
  selectionRefractoryMS : Constant  Value=selectionRefractoryMS
  seqReadyTime : Constant  Value=seqReadyTime
  seqRehearseTime : Constant  Value=seqRehearseTime
  sequenceMatrix : Constant  Value=sequenceMatrix
  showBackspace : Constant  Value=showBackspace
  showCueOffTarget : Constant  Value=showCueOffTarget
  showCueOnTarget : Constant  Value=showCueOnTarget
  showScores : Constant  Value=showScores
  showStartStop : Constant  Value=showStartStop
  showTargetText : Constant  Value=showTargetText
  showTypedText : Constant  Value=showTypedText
  showXYZaura : Constant  Value=showXYZaura
  soundOnError : Constant  Value=soundOnError
  soundOnFail : Constant  Value=soundOnFail
  soundOnGo : Constant  Value=soundOnGo
  soundOnOverTarget : Constant  Value=soundOnOverTarget
  soundOnSuccess : Constant  Value=soundOnSuccess
  splitDimensions : Constant  Value=splitDimensions
  stopOffTarget : Constant  Value=stopOffTarget
  stopOnClick : Constant  Value=stopOnClick
  targetDelay : Constant  Value=targetDelay
  targetDevice : Constant  Value=targetDevice
  targetDiameter : Constant  Value=targetDiameter
  targetDiameters : Constant  Value=targetDiameters
  targetInds : Constant  Value=targetInds
  targetRotDiameter : Constant  Value=targetRotDiameter
  targetSeq : Constant  Value=targetSeq
  targetSpaceX : Constant  Value=targetSpaceX
  targetSpaceY : Constant  Value=targetSpaceY
  taskType : Constant  Value=taskType
  trialTimeout : Constant  Value=trialTimeout
  trialsPerScore : Constant  Value=trialsPerScore
  useGloveLPF : Constant  Value=useGloveLPF
  useMouseLPF : Constant  Value=useMouseLPF
  useRandomDelay : Constant  Value=useRandomDelay
  vmrTheta : Constant  Value=vmrTheta
  whichMovements : Constant  Value=whichMovements
  workspaceR : Constant  Value=workspaceR
  workspaceR2 : Constant  Value=workspaceR2
  workspaceX : Constant  Value=workspaceX
  workspaceY : Constant  Value=workspaceY
  workspaceZ : Constant  Value=workspaceZ
  xk2DepthPos : Constant  Value=xk2DepthPos
  xk2DepthVel : Constant  Value=xk2DepthVel
  xk2HorizontalPos : Constant  Value=xk2HorizontalPos
  xk2HorizontalVel : Constant  Value=xk2HorizontalVel
  xk2Rotate2Pos : Constant  Value=xk2Rotate2Pos
  xk2Rotate2Vel : Constant  Value=xk2Rotate2Vel
  xk2RotatePos : Constant  Value=xk2RotatePos
  xk2RotateVel : Constant  Value=xk2RotateVel
  xk2VerticalPos : Constant  Value=xk2VerticalPos
  xk2VerticalVel : Constant  Value=xk2VerticalVel
  xkRawSpeedCap : Constant  Value=xkRawSpeedCap
  xpcVelocityOutputPeriodMS : Constant  Value=xpcVelocityOutputPeriodMS
  taskParamsBus : Outport
  wires:
  targetDiameter/1 -> BusOutput/1  "targetDiameter"
  maxTaskTime/1 -> BusOutput/2  "maxTaskTime"
  holdTime/1 -> BusOutput/3  "holdTime"
  trialTimeout/1 -> BusOutput/4  "trialTimeout"
  numTrials/1 -> BusOutput/5  "numTrials"
  randomSeed/1 -> BusOutput/6  "randomSeed"
  expRandMu/1 -> BusOutput/7  "expRandMu"
  expRandMin/1 -> BusOutput/8  "expRandMin"
  expRandMax/1 -> BusOutput/9  "expRandMax"
  expRandBinSize/1 -> BusOutput/10  "expRandBinSize"
  taskType/1 -> BusOutput/11  "taskType"
  targetInds/1 -> BusOutput/12  "targetInds"
  numTargets/1 -> BusOutput/13  "numTargets"
  gain/1 -> BusOutput/14  "gain"
  failurePenalty/1 -> BusOutput/15  "failurePenalty"
  cursorDiameter/1 -> BusOutput/16  "cursorDiameter"
  inputType/1 -> BusOutput/17  "inputType"
  gloveBias/1 -> BusOutput/18  "gloveBias"
  useRandomDelay/1 -> BusOutput/19  "useRandomDelay"
  mouseOffset/1 -> BusOutput/20  "mouseOffset"
  workspaceX/1 -> BusOutput/21  "workspaceX"
  workspaceY/1 -> BusOutput/22  "workspaceY"
  workspaceZ/1 -> BusOutput/23  "workspaceZ"
  workspaceR/1 -> BusOutput/24  "workspaceR"
  workspaceR2/1 -> BusOutput/25  "workspaceR2"
  showScores/1 -> BusOutput/26  "showScores"
  trialsPerScore/1 -> BusOutput/27  "trialsPerScore"
  cursorColorClick/1 -> BusOutput/28  "cursorColorClick"
  recenterOnFail/1 -> BusOutput/29  "recenterOnFail"
  recenterOnSuccess/1 -> BusOutput/30  "recenterOnSuccess"
  recenterDelay/1 -> BusOutput/31  "recenterDelay"
  initialInput/1 -> BusOutput/32  "initialInput"
  clickPercentage/1 -> BusOutput/33  "clickPercentage"
  lockFingerPosition/1 -> BusOutput/34  "lockFingerPosition"
  fingerPositionTolerance/1 -> BusOutput/35  "fingerPositionTolerance"
  failOnLiftoff/1 -> BusOutput/36  "failOnLiftoff"
  errorAssistR/1 -> BusOutput/37  "errorAssistR"
  errorAssistTheta/1 -> BusOutput/38  "errorAssistTheta"
  errorAssistAxis/1 -> BusOutput/39  "errorAssistAxis"
  useGloveLPF/1 -> BusOutput/40  "useGloveLPF"
  gloveLPNumerator/1 -> BusOutput/41  "gloveLPNumerator"
  gloveLPDenominator/1 -> BusOutput/42  "gloveLPDenominator"
  gloveNonlinearCorrection/1 -> BusOutput/43  "gloveNonlinearCorrection"
  gloveYCorrection/1 -> BusOutput/44  "gloveYCorrection"
  gloveXCorrection/1 -> BusOutput/45  "gloveXCorrection"
  useMouseLPF/1 -> BusOutput/46  "useMouseLPF"
  soundOnFail/1 -> BusOutput/47  "soundOnFail"
  soundOnGo/1 -> BusOutput/48  "soundOnGo"
  soundOnSuccess/1 -> BusOutput/49  "soundOnSuccess"
  soundOnOverTarget/1 -> BusOutput/50  "soundOnOverTarget"
  mouseLPNumerator/1 -> BusOutput/51  "mouseLPNumerator"
  mouseLPDenominator/1 -> BusOutput/52  "mouseLPDenominator"
  stopOffTarget/1 -> BusOutput/53  "stopOffTarget"
  stopOnClick/1 -> BusOutput/54  "stopOnClick"
  outputType/1 -> BusOutput/55  "outputType"
  xk2HorizontalPos/1 -> BusOutput/56  "xk2HorizontalPos"
  xk2HorizontalVel/1 -> BusOutput/57  "xk2HorizontalVel"
  xk2VerticalPos/1 -> BusOutput/58  "xk2VerticalPos"
  xk2VerticalVel/1 -> BusOutput/59  "xk2VerticalVel"
  xk2DepthPos/1 -> BusOutput/60  "xk2DepthPos"
  xk2DepthVel/1 -> BusOutput/61  "xk2DepthVel"
  xk2RotatePos/1 -> BusOutput/62  "xk2RotatePos"
  xk2RotateVel/1 -> BusOutput/63  "xk2RotateVel"
  xk2Rotate2Pos/1 -> BusOutput/64  "xk2Rotate2Pos"
  xk2Rotate2Vel/1 -> BusOutput/65  "xk2Rotate2Vel"
  gridEdges/1 -> BusOutput/66  "gridEdges"
  gridTilesEachDim/1 -> BusOutput/67  "gridTilesEachDim"
  selectionRefractoryMS/1 -> BusOutput/68  "selectionRefractoryMS"
  autoplayReactionTime/1 -> BusOutput/69  "autoplayReactionTime"
  autoplayMovementDuration/1 -> BusOutput/70  "autoplayMovementDuration"
  powerGain/1 -> BusOutput/71  "powerGain"
  powerGainUnityCrossing/1 -> BusOutput/72  "powerGainUnityCrossing"
  targetRotDiameter/1 -> BusOutput/73  "targetRotDiameter"
  autoplayRotationStart/1 -> BusOutput/74  "autoplayRotationStart"
  autoplayRotationDuration/1 -> BusOutput/75  "autoplayRotationDuration"
  randomTaskTargetDiameters/1 -> BusOutput/76  "randomTaskTargetDiameters"
  randomTaskTargetRotDiameters/1 -> BusOutput/77  "randomTaskTargetRotDiameters"
  randomTaskBoundaries/1 -> BusOutput/78  "randomTaskBoundaries"
  numDisplayDims/1 -> BusOutput/79  "numDisplayDims"
  cursorColorOpen/1 -> BusOutput/80  "cursorColorOpen"
  cursorColorClosed/1 -> BusOutput/81  "cursorColorClosed"
  showXYZaura/1 -> BusOutput/82  "showXYZaura"
  displayObject/1 -> BusOutput/83  "displayObject"
  preTrialLength/1 -> BusOutput/84  "preTrialLength"
  targetDiameters/1 -> BusOutput/85  "targetDiameters"
  numTargetDiameters/1 -> BusOutput/86  "numTargetDiameters"
  minTargetDistance/1 -> BusOutput/87  "minTargetDistance"
  targetDelay/1 -> BusOutput/88  "targetDelay"
  targetSpaceX/1 -> BusOutput/89  "targetSpaceX"
  targetSpaceY/1 -> BusOutput/90  "targetSpaceY"
  clickTargetColor/1 -> BusOutput/91  "clickTargetColor"
  clickTargetHoverColor/1 -> BusOutput/92  "clickTargetHoverColor"
  falseClickFails/1 -> BusOutput/93  "falseClickFails"
  splitDimensions/1 -> BusOutput/94  "splitDimensions"
  vmrTheta/1 -> BusOutput/95  "vmrTheta"
  xkRawSpeedCap/1 -> BusOutput/96  "xkRawSpeedCap"
  movementDuration/1 -> BusOutput/97  "movementDuration"
  holdDuration/1 -> BusOutput/98  "holdDuration"
  restDuration/1 -> BusOutput/99  "restDuration"
  returnDuration/1 -> BusOutput/100  "returnDuration"
  repsPerBlock/1 -> BusOutput/101  "repsPerBlock"
  whichMovements/1 -> BusOutput/102  "whichMovements"
  movementOrder/1 -> BusOutput/103  "movementOrder"
  delayOrder/1 -> BusOutput/104  "delayOrder"
  clickRefractoryPeriod/1 -> BusOutput/105  "clickRefractoryPeriod"
  xpcVelocityOutputPeriodMS/1 -> BusOutput/106  "xpcVelocityOutputPeriodMS"
  outputVelocityScaling/1 -> BusOutput/107  "outputVelocityScaling"
  screenUpdateRate/1 -> BusOutput/108  "screenUpdateRate"
  targetDevice/1 -> BusOutput/109  "targetDevice"
  playSpokenCues/1 -> BusOutput/110  "playSpokenCues"
  numTargetsInSeq/1 -> BusOutput/111  "numTargetsInSeq"
  targetSeq/1 -> BusOutput/112  "targetSeq"
  seqReadyTime/1 -> BusOutput/113  "seqReadyTime"
  seqRehearseTime/1 -> BusOutput/114  "seqRehearseTime"
  rotateSeqCues/1 -> BusOutput/115  "rotateSeqCues"
  numRepsPerSeq/1 -> BusOutput/116  "numRepsPerSeq"
  rehearsalOrder/1 -> BusOutput/117  "rehearsalOrder"
  rehearsalTimes/1 -> BusOutput/118  "rehearsalTimes"
  pathMode/1 -> BusOutput/119  "pathMode"
  memorizeMode/1 -> BusOutput/120  "memorizeMode"
  fixedSeqMode/1 -> BusOutput/121  "fixedSeqMode"
  sequenceMatrix/1 -> BusOutput/122  "sequenceMatrix"
  keyboard/1 -> BusOutput/123  "keyboard"
  resetDisplay/1 -> BusOutput/124  "resetDisplay"
  cursorNeuralColor/1 -> BusOutput/125  "cursorNeuralColor"
  cursorNonneuralColor/1 -> BusOutput/126  "cursorNonneuralColor"
  centerOffset/1 -> BusOutput/127  "centerOffset"
  scoreTime/1 -> BusOutput/128  "scoreTime"
  cuedTextLength/1 -> BusOutput/129  "cuedTextLength"
  cuedText/1 -> BusOutput/130  "cuedText"
  keyboardDims/1 -> BusOutput/131  "keyboardDims"
  recenterFullscreen/1 -> BusOutput/132  "recenterFullscreen"
  soundOnError/1 -> BusOutput/133  "soundOnError"
  acquireMethods/1 -> BusOutput/134  "acquireMethods"
  cumulativeDwell/1 -> BusOutput/135  "cumulativeDwell"
  showBackspace/1 -> BusOutput/136  "showBackspace"
  showStartStop/1 -> BusOutput/137  "showStartStop"
  showTargetText/1 -> BusOutput/138  "showTargetText"
  showTypedText/1 -> BusOutput/139  "showTypedText"
  showCueOnTarget/1 -> BusOutput/140  "showCueOnTarget"
  showCueOffTarget/1 -> BusOutput/141  "showCueOffTarget"
  recenterOffset/1 -> BusOutput/142  "recenterOffset"
  dwellRefractoryPeriod/1 -> BusOutput/143  "dwellRefractoryPeriod"
  keyPressedTime/1 -> BusOutput/144  "keyPressedTime"
  initialLockout/1 -> BusOutput/145  "initialLockout"
  initialState/1 -> BusOutput/146  "initialState"
  BusOutput/1 -> taskParamsBus/1

== matlab function keyboardTask/MATLAB Function ==
  data: taskParams input; keyboardOut output Bus: keysParamsBus; keyboard1 input Bus: keysParamsBus; keyboard2 input Bus: keysParamsBus; keyboard3 input; keyboard4 input; keyboard5 input; keyboard6 input; keyboard7 input; keyboard8 input; keyboard9 input; keyboard10 input; keyboard11 input; keyboard12 input; keyboard13 input; keyboard14 input; keyboard15 input; keyboard16 input; keyboard17 input; keyboard18 input; keyboard19 input
function keyboardOut = chooseKeyboard(taskParams, keyboard1, keyboard2, keyboard3, keyboard4, keyboard5, keyboard6, keyboard7, keyboard8, keyboard9, keyboard10, keyboard11, keyboard12, keyboard13, keyboard14, keyboard15, keyboard16, keyboard17, keyboard18, keyboard19)
%#codegen

switch taskParams.keyboard
    case uint16(keyboardConstants.KEYBOARD_QWERTY1)
        keyboardOut = keyboard1;
        
    case uint16(keyboardConstants.KEYBOARD_QWERTY2)
        keyboardOut = keyboard2;
        
    case uint16(keyboardConstants.KEYBOARD_GRID_6X6)
        keyboardOut = keyboard3;
        
    case uint16(keyboardConstants.KEYBOARD_GRID_7X7)
        keyboardOut = keyboard4;
        
    case uint16(keyboardConstants.KEYBOARD_GRID_8X8)
        keyboardOut = keyboard5;
        
    case uint16(keyboardConstants.KEYBOARD_GRID_9X9)
        keyboardOut = keyboard6;

    case uint16(keyboardConstants.KEYBOARD_GRID_10X10)
        keyboardOut = keyboard7;
    
    case uint16(keyboardConstants.KEYBOARD_QABCD)
        keyboardOut = keyboard8;

    case uint16(keyboardConstants.KEYBOARD_OPTIII)
        keyboardOut = keyboard9;

    case uint16(keyboardConstants.KEYBOARD_GRID_5X5)
        keyboardOut = keyboard10;

    case uint16(keyboardConstants.KEYBOARD_OPTIFREE)
        keyboardOut = keyboard11;        
        
    case uint16(keyboardConstants.KEYBOARD_GRID_12X12)
        keyboardOut = keyboard12;
        
    case uint16(keyboardConstants.KEYBOARD_GRID_14X14)
        keyboardOut = keyboard13;

    case uint16(keyboardConstants.KEYBOARD_GRID_15X15)
        keyboardOut = keyboard14;

    case uint16(keyboardConstants.KEYBOARD_GRID_16X16)
        keyboardOut = keyboard15;

    case uint16(keyboardConstants.KEYBOARD_GRID_18X18)
        keyboardOut = keyboard16;
        
    case uint16(keyboardConstants.KEYBOARD_GRID_20X20)
        keyboardOut = keyboard17;

    case uint16(keyboardConstants.KEYBOARD_GRID_22X22)
        keyboardOut = keyboard18;

    case uint16(keyboardConstants.KEYBOARD_GRID_24X24)
        keyboardOut = keyboard19;
        
        
    otherwise
        keyboardOut = keyboard1;
end
